simulink model "solar_collector_hot_water_storage_HE_zones"  (R2017a)
settings: Solver=VariableStepAuto  StartTime=0.0  StopTime=100000  RelTol=1e-3
values from neighbouring files (symbols this model uses):
  a1 = Ac*eta/C_c    (= 0.000575964912281)    [Linearized_model.m]    (also in Linearized_model_v1.m; Maple_linearization.m = 0.000380952380952; solar_collector_init.m = 7.33988724098e-05)
  a2 = -U_L1*Ac/2/C_c    (= -0.00145487240829)    [Linearized_model.m]    (also in Linearized_model_v1.m = -0.00290974481659; Maple_linearization.m = 0.00111111111111; solar_collector_init.m = -0.000214080044529)
  a3 = -U_L2*Ac/C_c    (= -7.48006379585e-06)    [Linearized_model.m]    (also in Linearized_model_v1.m; Maple_linearization.m = -0.00222222222222; solar_collector_init.m = 0.000428160089057)
  a4 = V_c^-1    (= 333.333333333)    [Linearized_model.m]    (also in Linearized_model_v1.m; Maple_linearization.m = 666.666666667; solar_collector_init.m = 133.333333333)
  a5 = -a4    (= -333.333333333)    [Linearized_model.m]    (also in Linearized_model_v1.m; Maple_linearization.m = -666.666666667; solar_collector_init.m = -133.333333333)
libraries: simulink x4
settings Model: Creator=info  LastModifiedBy=admin

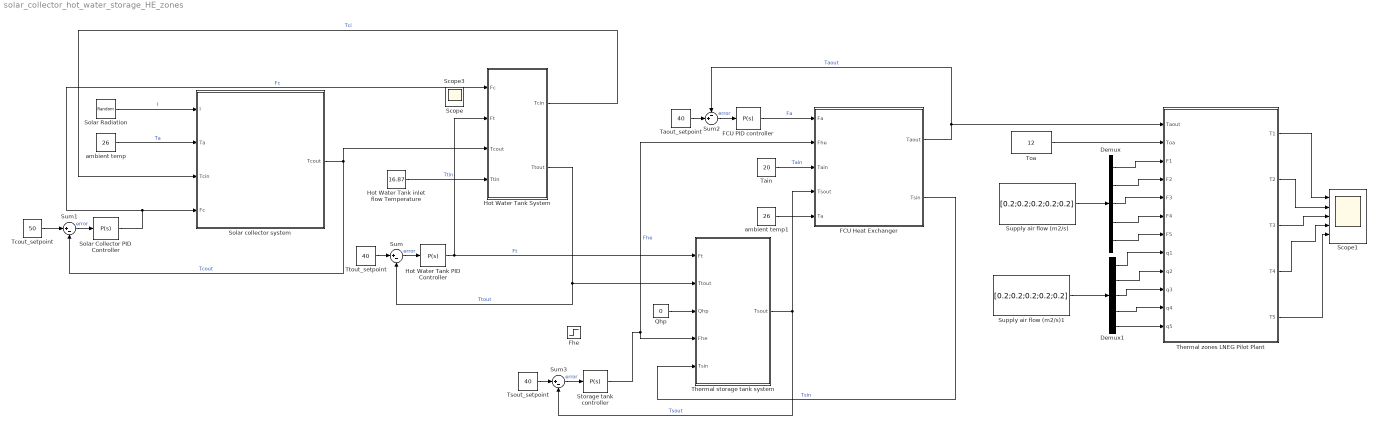
== system solar_collector_hot_water_storage_HE_zones ==
  Demux : Demux  Outputs=5
  Demux1 : Demux  Outputs=5
  FCU Heat Exchanger : Subsystem
      mask Display: image('heat_pump.PNG');
  "FCU PID controller " : simulink/Continuous/PID Controller  Controller=P  TimeDomain=Continuous-time  SampleTime=-1  IntegratorMethod=Forward Euler  FilterMethod=Forward Euler  Form=Parallel  UseFilter=on  ControllerParametersSource=internal  P=-0.0002  I=1.2  D=0.01  N=100  InitialConditionSource=internal  InitialConditionForIntegrator=0  InitialConditionForFilter=0  ExternalReset=none  ZeroCross=off  LimitOutput=on  UpperSaturationLimit=0.00015  LowerSaturationLimit=0  LinearizeAsGain=on  AntiWindupMode=none  Kb=1  TrackingMode=off  Kt=1  PParamMin=[]  PParamMax=[]  IParamMin=[]  IParamMax=[]  DParamMin=[]  DParamMax=[]  NParamMin=[]  NParamMax=[]  KbParamMin=[]  KbParamMax=[]  KtParamMin=[]  KtParamMax=[]  POutMin=[]  POutMax=[]  IOutMin=[]  IOutMax=[]  DOutMin=[]  DOutMax=[]  NOutMin=[]  NOutMax=[]  KbOutMin=[]  KbOutMax=[]  KtOutMin=[]  KtOutMax=[]  IntegratorOutMin=[]  IntegratorOutMax=[]  FilterOutMin=[]  FilterOutMax=[]  SumOutMin=[]  SumOutMax=[]  SumI1OutMin=[]  SumI1OutMax=[]  SumI2OutMin=[]  SumI2OutMax=[]  SumI3OutMin=[]  SumI3OutMax=[]  SumDOutMin=[]  SumDOutMax=[]  SaturationOutMin=[]  SaturationOutMax=[]  IntegratorContinuousStateAttributes=''  IntegratorStateMustResolveToSignalObject=off  IntegratorRTWStateStorageClass=Auto  FilterContinuousStateAttributes=''  FilterStateMustResolveToSignalObject=off  FilterRTWStateStorageClass=Auto  DifferentiatorICPrevScaledInput=0  DifferentiatorOutMin=[]  DifferentiatorOutMax=[]  InitialConditionSetting=State (most efficient)
  "Fhe " : Step  Time=5  After=0.000015  SampleTime=0
  Hot Water Tank PID Controller : simulink/Continuous/PID Controller  Controller=P  TimeDomain=Continuous-time  SampleTime=-1  IntegratorMethod=Forward Euler  FilterMethod=Forward Euler  Form=Parallel  UseFilter=on  ControllerParametersSource=internal  P=-0.0002  I=1.2  D=0.01  N=100  InitialConditionSource=internal  InitialConditionForIntegrator=0  InitialConditionForFilter=0  ExternalReset=none  ZeroCross=off  LimitOutput=on  UpperSaturationLimit=0.00015  LowerSaturationLimit=0  LinearizeAsGain=on  AntiWindupMode=none  Kb=1  TrackingMode=off  Kt=1  PParamMin=[]  PParamMax=[]  IParamMin=[]  IParamMax=[]  DParamMin=[]  DParamMax=[]  NParamMin=[]  NParamMax=[]  KbParamMin=[]  KbParamMax=[]  KtParamMin=[]  KtParamMax=[]  POutMin=[]  POutMax=[]  IOutMin=[]  IOutMax=[]  DOutMin=[]  DOutMax=[]  NOutMin=[]  NOutMax=[]  KbOutMin=[]  KbOutMax=[]  KtOutMin=[]  KtOutMax=[]  IntegratorOutMin=[]  IntegratorOutMax=[]  FilterOutMin=[]  FilterOutMax=[]  SumOutMin=[]  SumOutMax=[]  SumI1OutMin=[]  SumI1OutMax=[]  SumI2OutMin=[]  SumI2OutMax=[]  SumI3OutMin=[]  SumI3OutMax=[]  SumDOutMin=[]  SumDOutMax=[]  SaturationOutMin=[]  SaturationOutMax=[]  IntegratorContinuousStateAttributes=''  IntegratorStateMustResolveToSignalObject=off  IntegratorRTWStateStorageClass=Auto  FilterContinuousStateAttributes=''  FilterStateMustResolveToSignalObject=off  FilterRTWStateStorageClass=Auto  DifferentiatorICPrevScaledInput=0  DifferentiatorOutMin=[]  DifferentiatorOutMax=[]  InitialConditionSetting=State (most efficient)
  Hot Water Tank System : Subsystem
      mask Display: image('hot_water_tank.PNG');
  Hot Water Tank inlet flow Temperature : Constant  Value=16.87
  Qhp : Constant  Value=0
  Scope1 : Scope  NumInputPorts=5
  Solar Collector PID Controller : simulink/Continuous/PID Controller  Controller=P  TimeDomain=Continuous-time  SampleTime=-1  IntegratorMethod=Forward Euler  FilterMethod=Forward Euler  Form=Parallel  UseFilter=on  ControllerParametersSource=internal  P=-0.0002  I=1.2  D=0.01  N=100  InitialConditionSource=internal  InitialConditionForIntegrator=0  InitialConditionForFilter=0  ExternalReset=none  ZeroCross=off  LimitOutput=on  UpperSaturationLimit=0.00015  LowerSaturationLimit=0  LinearizeAsGain=on  AntiWindupMode=none  Kb=1  TrackingMode=off  Kt=1  PParamMin=[]  PParamMax=[]  IParamMin=[]  IParamMax=[]  DParamMin=[]  DParamMax=[]  NParamMin=[]  NParamMax=[]  KbParamMin=[]  KbParamMax=[]  KtParamMin=[]  KtParamMax=[]  POutMin=[]  POutMax=[]  IOutMin=[]  IOutMax=[]  DOutMin=[]  DOutMax=[]  NOutMin=[]  NOutMax=[]  KbOutMin=[]  KbOutMax=[]  KtOutMin=[]  KtOutMax=[]  IntegratorOutMin=[]  IntegratorOutMax=[]  FilterOutMin=[]  FilterOutMax=[]  SumOutMin=[]  SumOutMax=[]  SumI1OutMin=[]  SumI1OutMax=[]  SumI2OutMin=[]  SumI2OutMax=[]  SumI3OutMin=[]  SumI3OutMax=[]  SumDOutMin=[]  SumDOutMax=[]  SaturationOutMin=[]  SaturationOutMax=[]  IntegratorContinuousStateAttributes=''  IntegratorStateMustResolveToSignalObject=off  IntegratorRTWStateStorageClass=Auto  FilterContinuousStateAttributes=''  FilterStateMustResolveToSignalObject=off  FilterRTWStateStorageClass=Auto  DifferentiatorICPrevScaledInput=0  DifferentiatorOutMin=[]  DifferentiatorOutMax=[]  InitialConditionSetting=State (most efficient)
  Solar Radiation : RandomNumber  Mean=1360  Variance=0.5  SampleTime=0.1
  Solar collector system : Subsystem
      mask Display: image('collector_image.jpg');
  Storage tank controller : simulink/Continuous/PID Controller  Controller=P  TimeDomain=Continuous-time  SampleTime=-1  IntegratorMethod=Forward Euler  FilterMethod=Forward Euler  Form=Parallel  UseFilter=on  ControllerParametersSource=internal  P=0.002  I=1.2  D=0.01  N=100  InitialConditionSource=internal  InitialConditionForIntegrator=0  InitialConditionForFilter=0  ExternalReset=none  ZeroCross=off  LimitOutput=on  UpperSaturationLimit=0.00015  LowerSaturationLimit=0  LinearizeAsGain=on  AntiWindupMode=none  Kb=1  TrackingMode=off  Kt=1  PParamMin=[]  PParamMax=[]  IParamMin=[]  IParamMax=[]  DParamMin=[]  DParamMax=[]  NParamMin=[]  NParamMax=[]  KbParamMin=[]  KbParamMax=[]  KtParamMin=[]  KtParamMax=[]  POutMin=[]  POutMax=[]  IOutMin=[]  IOutMax=[]  DOutMin=[]  DOutMax=[]  NOutMin=[]  NOutMax=[]  KbOutMin=[]  KbOutMax=[]  KtOutMin=[]  KtOutMax=[]  IntegratorOutMin=[]  IntegratorOutMax=[]  FilterOutMin=[]  FilterOutMax=[]  SumOutMin=[]  SumOutMax=[]  SumI1OutMin=[]  SumI1OutMax=[]  SumI2OutMin=[]  SumI2OutMax=[]  SumI3OutMin=[]  SumI3OutMax=[]  SumDOutMin=[]  SumDOutMax=[]  SaturationOutMin=[]  SaturationOutMax=[]  IntegratorContinuousStateAttributes=''  IntegratorStateMustResolveToSignalObject=off  IntegratorRTWStateStorageClass=Auto  FilterContinuousStateAttributes=''  FilterStateMustResolveToSignalObject=off  FilterRTWStateStorageClass=Auto  DifferentiatorICPrevScaledInput=0  DifferentiatorOutMin=[]  DifferentiatorOutMax=[]  InitialConditionSetting=State (most efficient)
  Sum : Sum  Inputs=|+-
  Sum1 : Sum  Inputs=|+-
  Sum2 : Sum  Inputs=-+|
  Sum3 : Sum  Inputs=|+-
  Supply air flow (m2/s) : Constant  Value=[0.2;0.2;0.2;0.2;0.2]
  Supply air flow (m2/s)1 : Constant  Value=[0.2;0.2;0.2;0.2;0.2]
  Tain : Constant  Value=20
  Taout_setpoint : Constant  Value=40
  Tcout_setpoint : Constant  Value=50
  Thermal storage tank system : Subsystem
      mask Display: image('storage_tank.PNG');
  Thermal zones LNEG Pilot Plant : Subsystem
      mask Display: image('building.PNG');
  Toa : Constant  Value=12
  Tsout_setpoint : Constant  Value=40
  Ttout_setpoint : Constant  Value=40
  ambient temp : Constant  Value=26
  ambient temp1 : Constant  Value=26
  Scope : Scope
  Scope3 : Scope
  wires:
  Hot Water Tank System/1("Tcin ") -> Solar collector system/3(Tcin)  "Tci"
  ambient temp/1 -> Solar collector system/2(Ta)  "Ta"
  Solar Radiation/1 -> Solar collector system/1(I)  "I"
  Hot Water Tank System/2("Ttout ") -> Sum/2, Thermal storage tank system/2("Ttout ")  "Ttout"
  Ttout_setpoint/1 -> Sum/1
  Sum/1 -> Hot Water Tank PID Controller/1  "error"
  Solar Collector PID Controller/1 -> Hot Water Tank System/1("Fc "), Solar collector system/4(Fc)  "Fc"
  Hot Water Tank PID Controller/1 -> Hot Water Tank System/2(Ft), Thermal storage tank system/1("Ft ")  "Ft"
  Hot Water Tank inlet flow Temperature/1 -> Hot Water Tank System/4("Ttin ")  "Ttin"
  Sum1/1 -> Solar Collector PID Controller/1  "error"
  Tcout_setpoint/1 -> Sum1/1
  Solar collector system/1(Tcout) -> Sum1/2, Hot Water Tank System/3("Tcout ")  "Tcout"
  Qhp/1 -> Thermal storage tank system/3(Qhp)
  Thermal storage tank system/1("Tsout ") -> Sum3/2, FCU Heat Exchanger/4("Tsout ")  "Tsout"
  FCU Heat Exchanger/2("Tsin ") -> Thermal storage tank system/5(Tsin)  "Tsin"
  ambient temp1/1 -> FCU Heat Exchanger/5(Ta)
  Tain/1 -> FCU Heat Exchanger/3("Tain ")  "Tain"
  Storage tank controller/1 -> Thermal storage tank system/4(Fhe), FCU Heat Exchanger/2(Fhe)  "Fhe"
  Sum2/1 -> "FCU PID controller "/1  "error"
  Taout_setpoint/1 -> Sum2/2
  FCU Heat Exchanger/1("Taout ") -> Thermal zones LNEG Pilot Plant/1("Taout "), Sum2/1  "Taout"
  "FCU PID controller "/1 -> FCU Heat Exchanger/1("Fa ")  "Fa"
  Sum3/1 -> Storage tank controller/1  "error"
  Tsout_setpoint/1 -> Sum3/1
  Demux/4 -> Thermal zones LNEG Pilot Plant/6(F4)
  Demux/1 -> Thermal zones LNEG Pilot Plant/3("F1 ")
  Thermal zones LNEG Pilot Plant/1(T1) -> Scope1/1
  Demux1/1 -> Thermal zones LNEG Pilot Plant/8(q1)
  Supply air flow (m2/s)1/1 -> Demux1/1
  Thermal zones LNEG Pilot Plant/4(T4) -> Scope1/4
  Toa/1 -> Thermal zones LNEG Pilot Plant/2(Toa)
  Demux/3 -> Thermal zones LNEG Pilot Plant/5(F3)
  Supply air flow (m2/s)/1 -> Demux/1
  Thermal zones LNEG Pilot Plant/5(T5) -> Scope1/5
  Demux1/5 -> Thermal zones LNEG Pilot Plant/12(q5)
  Demux1/3 -> Thermal zones LNEG Pilot Plant/10(q3)
  Demux/2 -> Thermal zones LNEG Pilot Plant/4(F2)
  Demux1/4 -> Thermal zones LNEG Pilot Plant/11(q4)
  Thermal zones LNEG Pilot Plant/2(T2) -> Scope1/2
  Demux1/2 -> Thermal zones LNEG Pilot Plant/9(q2)
  Demux/5 -> Thermal zones LNEG Pilot Plant/7(F5)
  Thermal zones LNEG Pilot Plant/3(T3) -> Scope1/3

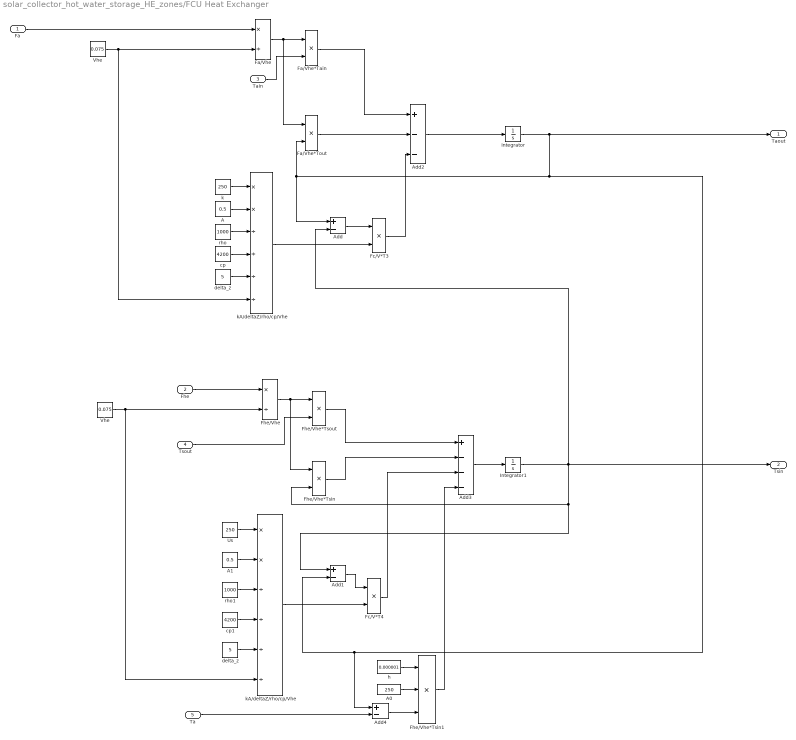
== system solar_collector_hot_water_storage_HE_zones/FCU Heat Exchanger ==
  "Fa " : Inport
  Fhe : Inport  Port=2
  "Tain " : Inport  Port=3
  "Tsout " : Inport  Port=4
  Ta : Inport  Port=5
  A : Constant  Value=0.5
  A0 : Constant  Value=250
  A1 : Constant  Value=0.5
  Add : Sum  Inputs=+-
  Add1 : Sum  Inputs=+-
  Add2 : Sum  Inputs=+--
  Add3 : Sum  Inputs=+---
  Add4 : Sum  Inputs=+-
  Fa/Vhe : Product  Inputs=*/
  Fa/Vhe*Tain : Product  Inputs=**
  Fa/Vhe*Tout : Product  Inputs=**
  Fc/V*T3 : Product  Inputs=**
  Fc/V*T4 : Product  Inputs=**
  Fhe/Vhe : Product  Inputs=*/
  Fhe/Vhe*Tsin : Product  Inputs=**
  Fhe/Vhe*Tsin1 : Product  Inputs=***
  Fhe/Vhe*Tsout : Product  Inputs=**
  Integrator : Integrator  InitialCondition=16.87
  Integrator1 : Integrator  InitialCondition=10
  "Us    " : Constant  Value=250
  Vhe : Constant  Value=0.075
  "Vhe " : Constant  Value=0.075
  cp : Constant  Value=4200
  cp1 : Constant  Value=4200
  delta_z : Constant  Value=5
  "delta_z " : Constant  Value=5
  h : Constant  Value=0.000001
  k : Constant  Value=250
  kA/deltaZ/rho/cp/Vhe : Product  Inputs=**////
  "kA/deltaZ/rho/cp/Vhe " : Product  Inputs=**////
  rho : Constant  Value=1000
  rho1 : Constant  Value=1000
  "Taout " : Outport
  "Tsin " : Outport  Port=2
  wires:
  Vhe/1 -> kA/deltaZ/rho/cp/Vhe/6, Fa/Vhe/2
  "Us    "/1 -> "kA/deltaZ/rho/cp/Vhe "/1
  Integrator1/1 -> Add1/1, Fhe/Vhe*Tsin/2, "Tsin "/1, Add/2
  "Tsout "/1 -> Fhe/Vhe*Tsout/2
  "Fa "/1 -> Fa/Vhe/1
  Fa/Vhe/1 -> Fa/Vhe*Tout/1, Fa/Vhe*Tain/1
  rho/1 -> kA/deltaZ/rho/cp/Vhe/3
  cp1/1 -> "kA/deltaZ/rho/cp/Vhe "/4
  A1/1 -> "kA/deltaZ/rho/cp/Vhe "/2
  Integrator/1 -> Add4/1, Add1/2, Fa/Vhe*Tout/2, Add/1, "Taout "/1
  k/1 -> kA/deltaZ/rho/cp/Vhe/1
  "Tain "/1 -> Fa/Vhe*Tain/2
  rho1/1 -> "kA/deltaZ/rho/cp/Vhe "/3
  Fhe/Vhe/1 -> Fhe/Vhe*Tsout/1, Fhe/Vhe*Tsin/1
  "Vhe "/1 -> "kA/deltaZ/rho/cp/Vhe "/6, Fhe/Vhe/2
  Fhe/1 -> Fhe/Vhe/1
  cp/1 -> kA/deltaZ/rho/cp/Vhe/4
  A/1 -> kA/deltaZ/rho/cp/Vhe/2
  Fa/Vhe*Tain/1 -> Add2/1
  Add2/1 -> Integrator/1
  kA/deltaZ/rho/cp/Vhe/1 -> Fc/V*T3/2
  Fc/V*T3/1 -> Add2/3
  Fhe/Vhe*Tsout/1 -> Add3/1
  Add3/1 -> Integrator1/1
  Add/1 -> Fc/V*T3/1
  Fa/Vhe*Tout/1 -> Add2/2
  Fhe/Vhe*Tsin/1 -> Add3/2
  Fc/V*T4/1 -> Add3/3
  "kA/deltaZ/rho/cp/Vhe "/1 -> Fc/V*T4/2
  Add1/1 -> Fc/V*T4/1
  delta_z/1 -> kA/deltaZ/rho/cp/Vhe/5
  "delta_z "/1 -> "kA/deltaZ/rho/cp/Vhe "/5
  Fhe/Vhe*Tsin1/1 -> Add3/4
  Ta/1 -> Add4/2
  Add4/1 -> Fhe/Vhe*Tsin1/3
  h/1 -> Fhe/Vhe*Tsin1/1
  A0/1 -> Fhe/Vhe*Tsin1/2

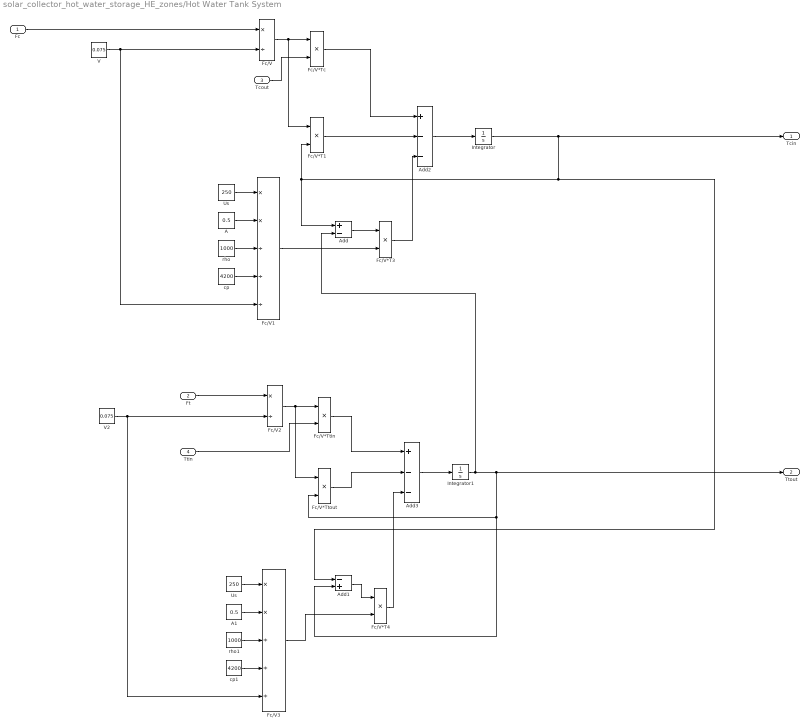
== system solar_collector_hot_water_storage_HE_zones/Hot Water Tank System ==
  "Fc " : Inport
  Ft : Inport  Port=2
  "Tcout " : Inport  Port=3
  "Ttin " : Inport  Port=4
  A : Constant  Value=0.5
  A1 : Constant  Value=0.5
  Add : Sum  Inputs=+-
  Add1 : Sum  Inputs=-+
  Add2 : Sum  Inputs=+--
  Add3 : Sum  Inputs=+--
  Fc/V : Product  Inputs=*/
  Fc/V*T1 : Product  Inputs=**
  Fc/V*T3 : Product  Inputs=**
  Fc/V*T4 : Product  Inputs=**
  Fc/V*Tc : Product  Inputs=**
  Fc/V*Ttin : Product  Inputs=**
  Fc/V*Ttout : Product  Inputs=**
  Fc/V1 : Product  Inputs=**///
  Fc/V2 : Product  Inputs=*/
  Fc/V3 : Product  Inputs=**///
  Integrator : Integrator  InitialCondition=16.87
  Integrator1 : Integrator  InitialCondition=10
  Us : Constant  Value=250
  "Us    " : Constant  Value=250
  V : Constant  Value=0.075
  V2 : Constant  Value=0.075
  cp : Constant  Value=4200
  cp1 : Constant  Value=4200
  rho : Constant  Value=1000
  rho1 : Constant  Value=1000
  "Tcin " : Outport
  "Ttout " : Outport  Port=2
  wires:
  V/1 -> Fc/V1/5, Fc/V/2
  "Us    "/1 -> Fc/V3/1
  Integrator1/1 -> Add1/2, Fc/V*Ttout/2, "Ttout "/1, Add/2
  "Ttin "/1 -> Fc/V*Ttin/2
  "Fc "/1 -> Fc/V/1
  Fc/V/1 -> Fc/V*T1/1, Fc/V*Tc/1
  rho/1 -> Fc/V1/3
  cp1/1 -> Fc/V3/4
  A1/1 -> Fc/V3/2
  Integrator/1 -> "Tcin "/1, Add1/1, Fc/V*T1/2, Add/1
  Us/1 -> Fc/V1/1
  "Tcout "/1 -> Fc/V*Tc/2
  rho1/1 -> Fc/V3/3
  Fc/V2/1 -> Fc/V*Ttin/1, Fc/V*Ttout/1
  V2/1 -> Fc/V2/2, Fc/V3/5
  Ft/1 -> Fc/V2/1
  cp/1 -> Fc/V1/4
  A/1 -> Fc/V1/2
  Fc/V*Tc/1 -> Add2/1
  Add2/1 -> Integrator/1
  Fc/V1/1 -> Fc/V*T3/2
  Fc/V*T3/1 -> Add2/3
  Fc/V*Ttin/1 -> Add3/1
  Add3/1 -> Integrator1/1
  Add/1 -> Fc/V*T3/1
  Fc/V*T1/1 -> Add2/2
  Fc/V*Ttout/1 -> Add3/2
  Fc/V*T4/1 -> Add3/3
  Fc/V3/1 -> Fc/V*T4/2
  Add1/1 -> Fc/V*T4/1

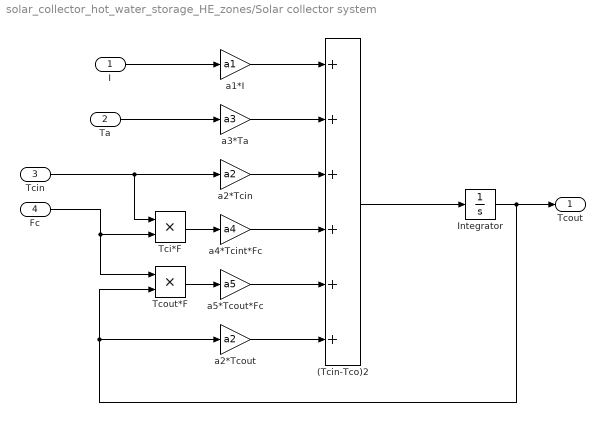
== system solar_collector_hot_water_storage_HE_zones/Solar collector system ==
  I : Inport
  Ta : Inport  Port=2
  Tcin : Inport  Port=3
  Fc : Inport  Port=4
  (Tcin-Tco)2 : Sum  Inputs=++++++
  Integrator : Integrator  InitialCondition=10
  Tci*F : Product  Inputs=**
  Tcout*F : Product  Inputs=**
  a1*I : Gain  Gain=a1
  a2*Tcin : Gain  Gain=a2
  "a2*Tcout " : Gain  Gain=a2
  a3*Ta : Gain  Gain=a3
  a4*Tcint*Fc : Gain  Gain=a4
  "a5*Tcout*Fc " : Gain  Gain=a5
  Tcout : Outport
  wires:
  I/1 -> a1*I/1
  Integrator/1 -> "a2*Tcout "/1, Tcout*F/2, Tcout/1
  (Tcin-Tco)2/1 -> Integrator/1
  Fc/1 -> Tcout*F/1, Tci*F/2
  a1*I/1 -> (Tcin-Tco)2/1
  Ta/1 -> a3*Ta/1
  Tcin/1 -> Tci*F/1, a2*Tcin/1
  a3*Ta/1 -> (Tcin-Tco)2/2
  a2*Tcin/1 -> (Tcin-Tco)2/3
  "a5*Tcout*Fc "/1 -> (Tcin-Tco)2/5
  Tci*F/1 -> a4*Tcint*Fc/1
  a4*Tcint*Fc/1 -> (Tcin-Tco)2/4
  Tcout*F/1 -> "a5*Tcout*Fc "/1
  "a2*Tcout "/1 -> (Tcin-Tco)2/6

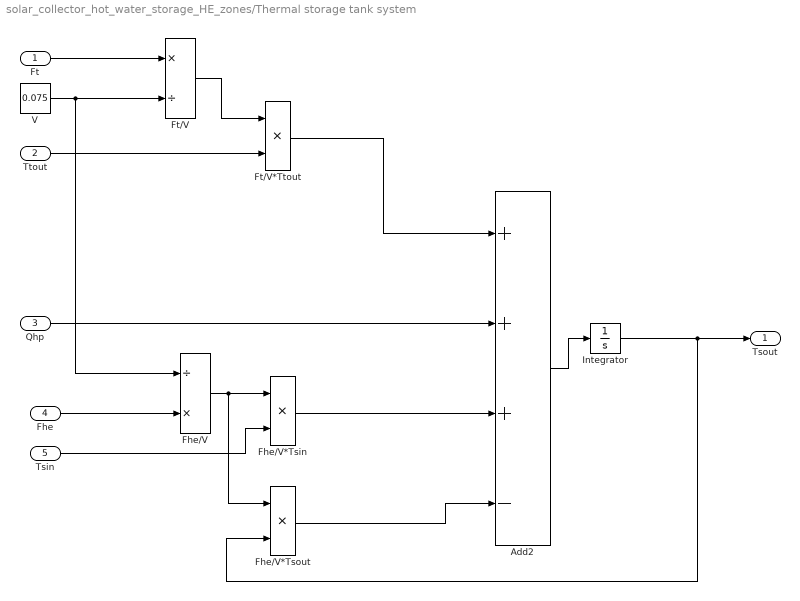
== system solar_collector_hot_water_storage_HE_zones/Thermal storage tank system ==
  "Ft " : Inport
  "Ttout " : Inport  Port=2
  Qhp : Inport  Port=3
  Fhe : Inport  Port=4
  Tsin : Inport  Port=5
  Add2 : Sum  Inputs=+++-
  Fhe/V : Product  Inputs=/*
  Fhe/V*Tsin : Product  Inputs=**
  Fhe/V*Tsout : Product  Inputs=**
  Ft/V : Product  Inputs=*/
  Ft/V*Ttout : Product  Inputs=**
  Integrator : Integrator  InitialCondition=16.87
  V : Constant  Value=0.075
  "Tsout " : Outport
  wires:
  "Ft "/1 -> Ft/V/1
  Ft/V/1 -> Ft/V*Ttout/1
  Integrator/1 -> "Tsout "/1, Fhe/V*Tsout/2
  "Ttout "/1 -> Ft/V*Ttout/2
  Ft/V*Ttout/1 -> Add2/1
  Add2/1 -> Integrator/1
  Tsin/1 -> Fhe/V*Tsin/2
  Fhe/V/1 -> Fhe/V*Tsout/1, Fhe/V*Tsin/1
  Fhe/V*Tsin/1 -> Add2/3
  V/1 -> Fhe/V/1, Ft/V/2
  Fhe/1 -> Fhe/V/2
  Qhp/1 -> Add2/2
  Fhe/V*Tsout/1 -> Add2/4

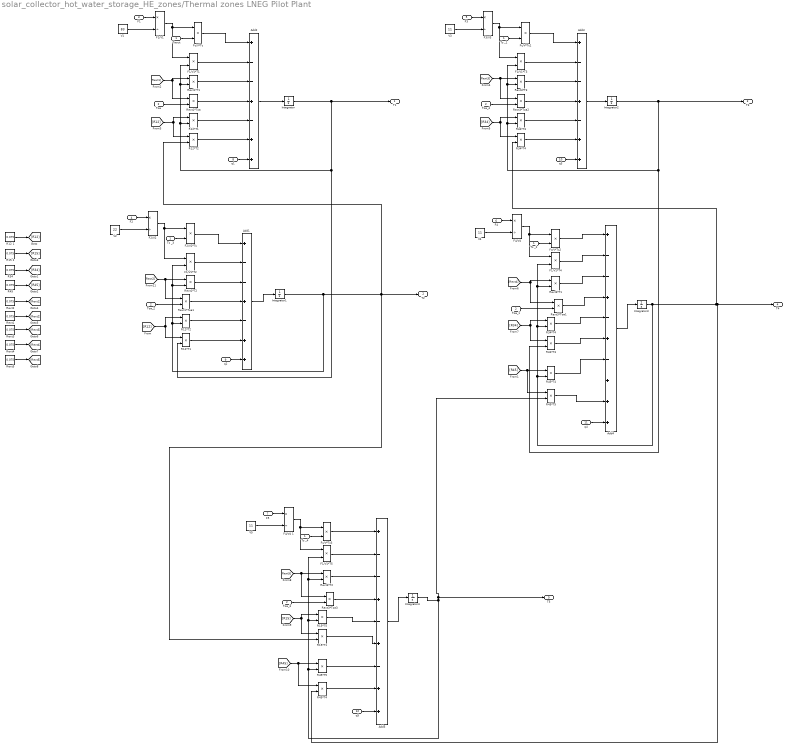
== system solar_collector_hot_water_storage_HE_zones/Thermal zones LNEG Pilot Plant ==
  "Taout " : Inport
  Toa : Inport  Port=2
  "F1 " : Inport  Port=3
  F2 : Inport  Port=4
  F3 : Inport  Port=5
  F4 : Inport  Port=6
  F5 : Inport  Port=7
  q1 : Inport  Port=8
  q2 : Inport  Port=9
  q3 : Inport  Port=10
  q4 : Inport  Port=11
  q5 : Inport  Port=12
  Add1 : Sum  Inputs=+--+-++
  Add2 : Sum  Inputs=+--+-++
  Add3 : Sum  Inputs=+--+-++
  Add4 : Sum  Inputs=+--+-+-+++
  Add5 : Sum  Inputs=+--+-+-++
  F1/V1 : Product  Inputs=*/
  F1/V1*T{1..5} (5 alike) : Product  Inputs=**
  F2/V2 : Product  Inputs=*/
  F2/V2*Ts : Product  Inputs=**
  F3/V3 : Product  Inputs=*/
  "F4/V4 " : Product  Inputs=*/
  F4/V4 1 : Product  Inputs=*/
  Fc/V*Tc{,1..3} (4 alike) : Product  Inputs=**
  Integrator{,1..4} (5 alike) : Integrator  InitialCondition=16.87
  R12 1 : Constant  Value=0.075
  R12*T1 : Product  Inputs=**
  "R12*T1 " : Product  Inputs=**
  R12*T2 : Product  Inputs=**
  "R12*T2 " : Product  Inputs=**
  R15 2 : Constant  Value=0.075
  R15*T1 : Product  Inputs=**
  R15*T5 : Product  Inputs=**
  "R34 " : Constant  Value=0.075
  R34*T3 : Product  Inputs=**
  "R34*T3  " : Product  Inputs=**
  R34*T4 : Product  Inputs=**
  "R34*T4   " : Product  Inputs=**
  "R45 " : Constant  Value=0.075
  R45*T4 : Product  Inputs=**
  "R45*T4      " : Product  Inputs=**
  R45*T5 : Product  Inputs=**
  "R45*T5    " : Product  Inputs=**
  Rext{1..5} (5 alike) : Constant  Value=0.075
  Rext1*T1 : Product  Inputs=**
  Rext1*T2 : Product  Inputs=**
  Rext1*Toa : Product  Inputs=**
  Rext1*Toa1 : Product  Inputs=**
  Rext3*T1 : Product  Inputs=**
  Rext3*T2 : Product  Inputs=**
  Rext3*T3 : Product  Inputs=**
  Rext3*Toa1 : Product  Inputs=**
  Rext3*Toa2 : Product  Inputs=**
  Rext3*Toa3 : Product  Inputs=**
  Toa_{1..4} (4 alike) : InportShadow  Port=2
  Ts _{1..4} (4 alike) : InportShadow
  V1 : Constant  Value=83
  V2 : Constant  Value=22
  V3 : Constant  Value=11
  V4 : Constant  Value=11
  V5 : Constant  Value=11
  T1 : Outport
  T2 : Outport  Port=2
  T3 : Outport  Port=3
  T4 : Outport  Port=4
  T5 : Outport  Port=5
  wires:
  Add3/1 -> Integrator2/1
  Ts _1/1 -> Fc/V*Tc1/2
  Toa_4/1 -> Rext3*Toa2/2
  R34*T4/1 -> Add3/6
  V3/1 -> F3/V3/2
  Fc/V*Tc1/1 -> Add3/1
  Rext3*T3/1 -> Add3/3
  F1/V1*T3/1 -> Add3/2
  Rext3*Toa2/1 -> Add3/4
  Integrator2/1 -> T3/1, "R34*T3  "/2, R34*T3/2, Rext3*T3/2, F1/V1*T3/2
  F3/1 -> F3/V3/1
  q3/1 -> Add3/7
  R34*T3/1 -> Add3/5
  [R34] -> R34*T4/1, R34*T3/1
  F3/V3/1 -> F1/V1*T3/1, Fc/V*Tc1/1
  [Rext3] -> Rext3*Toa2/1, Rext3*T3/1
  q5/1 -> Add5/9
  R12 1/1 -> [R12]
  Rext3*T2/1 -> Add5/3
  R15*T5/1 -> Add5/5
  R15*T1/1 -> Add5/6
  R45*T5/1 -> Add5/7
  Ts _4/1 -> Fc/V*Tc3/2
  [R45] -> R45*T4/1, R45*T5/1
  Rext3*Toa3/1 -> Add5/4
  F4/V4 1/1 -> F1/V1*T5/1, Fc/V*Tc3/1
  Add5/1 -> Integrator4/1
  Toa_3/1 -> Rext3*Toa3/2
  V5/1 -> F4/V4 1/2
  F1/V1*T5/1 -> Add5/2
  F5/1 -> F4/V4 1/1
  [R15] -> R15*T1/1, R15*T5/1
  [Rext5] -> Rext3*Toa3/1, Rext3*T2/1
  Fc/V*Tc3/1 -> Add5/1
  R15 2/1 -> [R15]
  Rext2/1 -> [Rext1]
  Rext3/1 -> [Rext3]
  Rext1/1 -> [Rext2]
  Rext4/1 -> [Rext4]
  Rext5/1 -> [Rext5]
  [R45] -> "R45*T5    "/1, "R45*T4      "/1
  "R45*T4      "/1 -> Add4/7
  Toa/1 -> Rext1*Toa/2
  q1/1 -> Add2/7
  Integrator/1 -> T1/1, "R12*T1 "/2, R12*T1/2, Rext1*T1/2, F1/V1*T1/2
  F1/V1/1 -> F1/V1*T1/1, Fc/V*Tc/1
  V1/1 -> F1/V1/2
  Add2/1 -> Integrator/1
  "F1 "/1 -> F1/V1/1
  Fc/V*Tc/1 -> Add2/1
  F1/V1*T1/1 -> Add2/2
  "Taout "/1 -> Fc/V*Tc/2
  R12*T1/1 -> Add2/5
  R12*T2/1 -> Add2/6
  [R12] -> R12*T2/1, R12*T1/1
  Rext1*Toa/1 -> Add2/4
  V2/1 -> F2/V2/2
  Toa_2/1 -> Rext1*Toa1/2
  F2/V2*Ts/1 -> Add1/1
  Rext1*Toa1/1 -> Add1/4
  q2/1 -> Add1/7
  F2/V2/1 -> F1/V1*T2/1, F2/V2*Ts/1
  Ts _3/1 -> F2/V2*Ts/2
  [R12] -> "R12*T1 "/1, "R12*T2 "/1
  Integrator1/1 -> T2/1, R15*T1/2, R12*T2/2, "R12*T2 "/2, Rext1*T2/2, F1/V1*T2/2
  Rext1*T2/1 -> Add1/3
  [Rext2] -> Rext1*Toa1/1, Rext1*T2/1
  "R12*T2 "/1 -> Add1/5
  "R12*T1 "/1 -> Add1/6
  F2/1 -> F2/V2/1
  Add1/1 -> Integrator1/1
  Rext1*T1/1 -> Add2/3
  F1/V1*T2/1 -> Add1/2
  [Rext1] -> Rext1*Toa/1, Rext1*T1/1
  "R45*T5    "/1 -> Add4/9
  R45*T4/1 -> Add5/8
  Integrator4/1 -> "R45*T5    "/2, T5/1, R45*T5/2, R15*T5/2, Rext3*T2/2, F1/V1*T5/2
  q4/1 -> Add4/10
  Integrator3/1 -> R34*T4/2, T4/1, R45*T4/2, "R45*T4      "/2, "R34*T4   "/2, Rext3*T1/2, F1/V1*T4/2
  F1/V1*T4/1 -> Add4/2
  Rext3*T1/1 -> Add4/3
  V4/1 -> "F4/V4 "/2
  Fc/V*Tc2/1 -> Add4/1
  "R34*T4   "/1 -> Add4/5
  Rext3*Toa1/1 -> Add4/4
  Add4/1 -> Integrator3/1
  F4/1 -> "F4/V4 "/1
  Toa_1/1 -> Rext3*Toa1/2
  [R34] -> "R34*T3  "/1, "R34*T4   "/1
  "R34*T3  "/1 -> Add4/6
  "F4/V4 "/1 -> F1/V1*T4/1, Fc/V*Tc2/1
  Ts _2/1 -> Fc/V*Tc2/2
  [Rext4] -> Rext3*Toa1/1, Rext3*T1/1
  "R45 "/1 -> [R45]
  "R34 "/1 -> [R34]
